simulink model "pemfc_lumpekf2_prerun"  (R2020b)
settings: Solver=VariableStepAuto  StartTime=0.0  StopTime=tend  MaxStep=dt  RelTol=1e-3
values from neighbouring files (symbols this model uses):
  P0 = diag([10,10,10000,10000,10000])    [input_sine.m]    (also in input_step.m)
  Qsys = diag([0.1^2 0.021^2 0.1^2/Area^2])    [input_sine.m]    (also in input_step.m; run_pemfc_lumpekf2.m = diag([diag(Qsys);0.01*param.Ndot_a;0.01*param.Ndot_c]))
  Rsys = 0.1^2    (= 0.01)    [input_sine.m]    (also in input_step.m)
  xhat0 = [0;0;0;0;0]    [input_sine.m]    (also in input_step.m)
undefined symbols (not defined in the file or in its folder): param
settings Model: Creator=kvijayar  LastModifiedBy=kvijayar

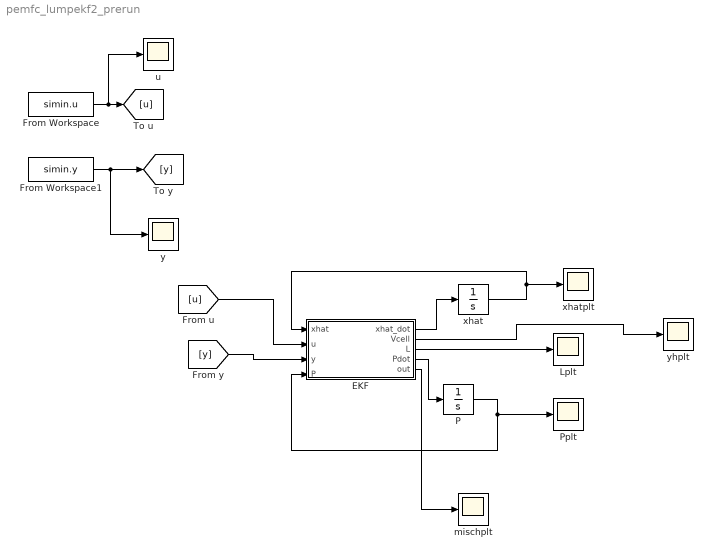
== system pemfc_lumpekf2_prerun ==
  EKF : MATLAB Function  TreatAsAtomicUnit=on
  From Workspace : FromWorkspace  VariableName=simin.u  OutputAfterFinalValue=Holding final value
  From Workspace1 : FromWorkspace  VariableName=simin.y  OutputAfterFinalValue=Holding final value
  Lplt : Scope
  P : Integrator  InitialCondition=P0
  Pplt : Scope
  mischplt : Scope
  u : Scope
  xhat : Integrator  InitialCondition=xhat0
  xhatplt : Scope
  y : Scope
  yhplt : Scope
  wires:
  EKF/4(Pdot) -> P/1
  P/1 -> Pplt/1, EKF/4(P)
  EKF/3(L) -> Lplt/1
  From Workspace1/1 -> y/1, [y]
  [y] -> EKF/3(y)
  EKF/1(xhat_dot) -> xhat/1
  xhat/1 -> EKF/1(xhat), xhatplt/1
  EKF/5(out) -> mischplt/1
  From Workspace/1 -> u/1, [u]
  [u] -> EKF/2(u)
  EKF/2(Vcell) -> yhplt/1

== matlab function pemfc_lumpekf2_prerun/EKF ==
  data: xhat_dot output; Vcell output; xhat input; u input; y input; L output; P input; Pdot output; Rsys parameter; Qsys parameter; param parameter; out output
function [xhat_dot,Vcell, L,Pdot,out] = EKF(xhat,u,y, P,Rsys,Qsys, param)

    x = xhat;
    phiH2_in=u(1); phiO2_in=u(2); J_in=u(3); Ndot_a=u(4); Ndot_c=u(5);

%%Common
    %x=[ϕ_0,ϕ_1,J_0,J_1,J_act ]^T --> change J to current?; u(1),u(2),ϕ_0,ϕ_1 are partial presure
    %u = [ϕ_(H2,A)^in, ϕ_(o2,C)^in, J]';
    %τ_m=1/(Dλ_m^2 )=τ_0/(2m+1)^2 
    tau0_1 = 1/param.tau_flux_O2;
    tau1_1 = 9*tau0_1; %tau0/(2*1+1)^2
    J_act = x(5);
    Area = param.lc*param.w;
    I = J_in*Area;
    %tauact = √(4J_0^2+(J_act )^2 )/(2V_(act,0) C_DL/Area)
    tauact_1 = Area*sqrt( 4*param.BV_J0^2 + J_act^2 )/( 2*param.BV_Vact0*param.Cdbl );
    tauactH2_1 = Area*sqrt( 4*param.BV_JH20^2 + J_act^2 )/( 2*param.BV_VactH20*param.Cdbl );
    
    %[4J_0^2+2J_act^2-J J_act ]/(4J_0^2+J_act^2 )
    tauact_ekf= tauact_1*( 4*param.BV_J0^2 + 2*J_act^2 - J_in*J_act)/( 4*param.BV_J0^2 + J_act^2 );
    tauactH2_ekf=tauactH2_1*( 4*param.BV_JH20^2 + 2*J_act^2 - J_in*J_act)/( 4*param.BV_JH20^2 + J_act^2 );
    %%EKF
    %f=param.ekf.f;
    Tch=( 0.1512*J_in + 4/pi*x(3) - 4/(3*pi)*x(4) )*Area/(4*param.Ndot_c*param.F); %Γ_ch≔J̅/nF --> (J̅A)⁄(4Ṅ_C F)
    phiO2_out = param.Pc - (param.Pc-phiO2_in)/(1-Tch);
    if param.ekf.f >= 0
        f=param.ekf.f;
    else
        if (phiO2_out>0)
            f=0.5;
        else
            %Find at what what point in channel phiO2_out=0
            %(Tch) = (phiO2_in/param.Pc);
            %phi_avg = f*phiO2_in+(1-f)*phiO2_out; --> f % of inlet in blend
            fend=phiO2_in/param.Pc/Tch;
            f=fend/2;
        end
    end
    L_zFD=param.xO2normal/param.J_lim;
    
    h_H2=(1-f*J_in*Area/(2*Ndot_a*param.F))/(1-J_in*Area/(2*Ndot_a*param.F));
    h_H2J=(1-f)*(param.Pc-phiH2_in)/(1-J_in*Area/(2*Ndot_a*param.F))^2*Area/(2*Ndot_a*param.F);
    h_H2N=h_H2J*J_in/Ndot_a;
    
    %0.1512J_act+4/π J_0-4/3π J_1
    Jbar=0.1512*x(5)+4/pi*x(3)-4/(3*pi)*x(4);
    %h_O2=(1-f (J ̅A)⁄(4N ̇_C param.F))/(1-(J ̅A)⁄(4N ̇_C param.F)),
    h_O2=(1-f*Jbar*Area/(4*Ndot_c*param.F))/(1-Jbar*Area/(4*Ndot_c*param.F));
    %h_O2J=(1-f)(P_A-ϕ_(O2,C)^in )/(1-(J ̅A)⁄(4N ̇_C param.F))^2   Area/(4N ̇_C param.F),
    h_O2J=(1-f)*(param.Pa-phiO2_in)/(1-Jbar*Area/(4*Ndot_c*param.F))^2*Area/(4*Ndot_c*param.F);
    %h_O2N=(h_O2J J ̅)/N ̇_C
    h_O2N=h_O2J*Jbar/Ndot_c;

    phiO2_1.MO2avg=0.1512*h_O2J *[0 0 4/pi -4/(3*pi) 0.1512];
    phiO2_1.MO2avgU = [0 h_O2 0 0 h_O2N];
    phiO2_0.MO2avg=zeros(1,5);
    phiO2_0.MO2avgU = [0 f 0 0 0];
    if phiO2_out > param.sim.phiO2_eps
        f_ = 1;
    else
        if phiO2_out < 0
            phiO2_out = 0;
        end
        f_ = phiO2_out/param.sim.phiO2_eps;
    end
    MO2avg=f_*phiO2_1.MO2avg + (1-f_)*phiO2_0.MO2avg;
    MO2avgU=f_*phiO2_1.MO2avgU + (1-f_)*phiO2_0.MO2avgU;

    phi_avg = f*phiO2_in+(1-f)*phiO2_out;
        
    MO2eff= MO2avg+[4/pi -4/(3*pi) -8/pi^2*L_zFD 0 -0.1894*L_zFD];
    MO2effU=0.1512*MO2avgU;

    %ϕ_(O2,eff)=[0.1512×ϕ_(O2-ch)-4/π ϕ_0+4/3π ϕ_1 ]-[0.1894J-8/π^2  J_0 ]×L/zFD
    %Assume phi_nom - Jlim*L/(zFD) = 0 OR L/(zFD) = phi_nom/J_lim
    phi_eff = 0.1512*phi_avg + 4/pi*x(1) - 4/(3*pi)*x(2) ...
        - (0.1894*J_in + 8/pi^2*x(3))*L_zFD;
    Vohm = (param.r1*I+ param.r2*I^2 - param.rt*(param.Tfc-298)*I);  

%% EKF A,B,C,D
    %Non-zero
    phieff_1.A=...
		 -diag([tau0_1,tau1_1,tau0_1,tau1_1,tauact_ekf])...
            +[zeros(5,4),[0;0;tau0_1;tau1_1;0]]...
            +[tau0_1*MO2avg;tau1_1*MO2avg;zeros(3,5)];
    phieff_1.B=...
		[ tau0_1*MO2avgU;
            tau1_1*MO2avgU;
            0   0   0   0   0;
            0   0   0   0   0;
            0   0   tauact_1    0   0];
    phieff_1.C=param.Bconc*phi_eff*MO2eff...
            -2*param.BV_Vact0/sqrt( 4*param.BV_J0^2 + J_act^2 )*[0 0 0 0 1];
    phieff_1.D=2*param.Bconc/(phiH2_in)*[h_H2 0 h_H2J -h_H2N 0]...
            + param.Bconc/(phi_eff)*MO2effU...
            + [0 0 -(param.r1+ param.r2*I - param.rt*(param.Tfc-298))*Area 0 0];
    phieff_1.Vact=2*param.BV_Vact0*asinh(J_act*Area/(2*param.BV_I0));
    phieff_1.Ecellc=0;
    %phieff_1.Ecellc=param.E0_cell;% - param.kE*(param.Tfc-298) ...
    %       + 2*param.Bconc*log(phiH2_in) + param.Bconc*log(phi_eff) ;
    
    %Zero
    phieff_0.A=-diag([tau0_1,tau1_1,tau0_1,tau1_1,tauactH2_1])...
            +[zeros(5,4),[0;0;tau0_1;tau1_1;0]];
    phieff_0.B=...
		[ tau0_1*MO2avgU;
            tau1_1*MO2avgU;
            0   0   0   0   0;
            0   0   0   0   0;
            0   0   tauactH2_ekf    0   0];
    phieff_0.C=-2*param.BV_VactH20/sqrt( 4*param.BV_JH20^2 + J_act^2 )*[0 0 0 0 1];
    phieff_0.D=[0 0 -(param.r1+ param.r2*I - param.rt*(param.Tfc-298))*Area 0 0];
    phieff_0.Vact=...
		 2*param.BV_VactH20*asinh(J_act/(2*param.BV_JH20));
    phieff_0.Ecellc=0;
    if phi_eff > param.sim.phieff_eps
        phieff.f = 1;
    else
        if phi_eff < 0
            phi_eff = 0;
        end
        phieff.f = phi_eff/param.sim.phieff_eps;
    end
    %y = 0.5*param.Bconc*log(phi_eff) - 2*param.BV_Vact0*asinh(J_act*Area/(2*param.BV_I0));
    %Vcell = Ecellc - Vohm - Vact;
%% Cell output
    %%System x dot
    E0T = param.E0_cell - param.kE*(param.Tfc-298);
    %phi_eff > 0
    phieff_1.dx = [
        tau0_1*( phi_avg - x(1) );
        tau1_1*( phi_avg - x(2) );
        tau0_1*( x(5) - x(3) );
        tau1_1*( x(5) - x(4) );
        tauact_1*( J_in - x(5) )
    ];
    phieff_1.Vact = 2*param.BV_Vact0*asinh(J_act/(2*param.BV_J0));
    if (phi_eff > 0)
        phieff_1.Econc = 2*param.Bconc*log(phiH2_in) + param.Bconc*log(phi_eff);
        phieff_1.Ecellc =  E0T +  phieff_1.Econc;
        if (phieff_1.Ecellc<0)
            phieff_1.Ecellc = 0;
            phieff_1.Econc = -E0T;
        end
    else
            phieff_1.Ecellc = 0;
            phieff_1.Econc = -E0T;    
    end

    %phi_eff <= 0
    phieff_0.dx = [
        tau0_1*( phi_avg - x(1) );
        tau1_1*( phi_avg - x(2) );
        tau0_1*( x(5) - x(3) );
        tau1_1*( x(5) - x(4) );
        tauactH2_1*( J_in - x(5) )
    ];
    phieff_0.Vact = 2*param.BV_VactH20*asinh(J_act/(2*param.BV_JH20));
    phieff_0.Ecellc = 0;
    phieff_0.E0T = param.E0_cell - param.kE*(param.Tfc-298);
    phieff_0.Econc=-E0T;  
    
%% Final
    %EKF
    f_=phieff.f;
    A = f_*phieff_1.A + (1-f_)*phieff_0.A;
    B = f_*phieff_1.B + (1-f_)*phieff_0.B;
    C = f_*phieff_1.C + (1-f_)*phieff_0.C;
    D = f_*phieff_1.D + (1-f_)*phieff_0.D;

    Qb = B*Qsys*B';
    Rb = Rsys+D*Qsys*D';
    %t = P*C';t = P*C'*(Rb)^-1;
    Pdot = A*P+P*A'-P*C'*(Rb)^-1*C*P+Qb;
    L = P*C';
    L = P*C'*(Rb)^-1;
    
    %Cell output
    
    Econc = f_*phieff_1.Econc + (1-f_)*phieff_0.Econc;
    Ecellc = f_*phieff_1.Ecellc + (1-f_)*phieff_0.Ecellc;
    Vact = f_*phieff_1.Vact + (1-f_)*phieff_0.Vact;
    dx = f_*phieff_1.dx + (1-f_)*phieff_0.dx;
    Vcell = Ecellc - Vohm - Vact;
    xhat_dot = dx + L*(y-Vcell);
    out = [phi_eff,phi_avg,phiO2_out,Ecellc,Vohm,Vact,E0T,Econc];
    %out.phi_eff = phi_eff;
